simulink model "cv_model_50M"  (R2023a)
settings: Solver=ode23t  StartTime=0  StopTime=5040  FixedStep=0.0005  MaxStep=.01  RelTol=1e-4
model workspace (MAT data in the model file):
  test = 0
values from neighbouring files (symbols this model uses):
  A_cheb_09_1 = [-9.45889157397 1 0 0 0 0 0 0 0 -116.684730988 0 1 ... (81 elements, 9x9)]    [input_reflex_filters.mat]
  B_cheb_09_1 = [1 0 0 0 0 0 0 0 0]    [input_reflex_filters.mat]
  C_cheb_09_1 = [0 0 0 0 0 0 0 0 151338.279895]    [input_reflex_filters.mat]
libraries: SignalEditorBlockLib x4, simulink_extras x2
(part 3 of 3)

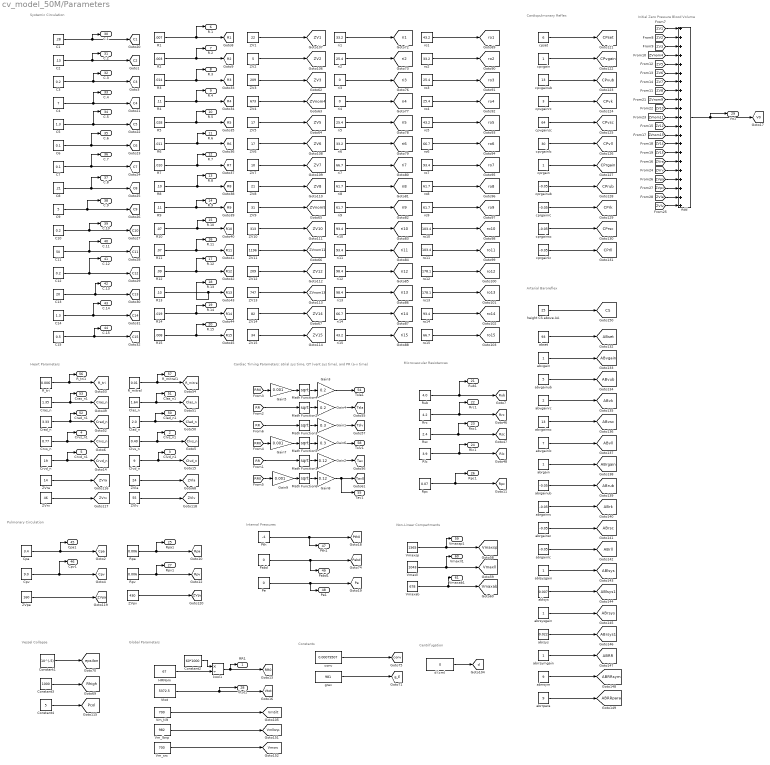
== system cv_model_50M/Parameters ==
  note: Initial Zero Pressure Blood Volume
  note: Cardiopulmonary Reflex
  note: Centrifugation
  note: Constants
  note: Vessel Collapse
  note: Non-Linear Compartments
  note: Heart Parameters
  note: Cardiac Timing Parameters: atrial sys time, QT (vent sys time), and PR (a-v time)
  note: Internal Pressures
  note: Pulmonary Circulation
  note: Microvascular Resistances
  note: Global Parameters
  note: Systemic Circulation
  note: Arterial Baroreflex
  Add : Sum  Inputs=+++++++++++++++++++++
  C1 : Constant  Value=.28
  C10 : Constant  Value=0.2
  C11 : Constant  Value=50
  C12 : Constant  Value=0.2
  C13 : Constant  Value=20
  C14 : Constant  Value=1.3
  C15 : Constant  Value=0.5
  C2 : Constant  Value=.13
  C3 : Constant  Value=0.2
  C4 : Constant  Value=7
  C5 : Constant  Value=1.3
  C6 : Constant  Value=0.1
  C7 : Constant  Value=0.1
  C8 : Constant  Value=.21
  C9 : Constant  Value=5
  Clad_n : Constant  Value=2.0
  Clas_n : Constant  Value=1.64
  Clvd_n : Constant  Value=9
  Clvs_n : Constant  Value=0.40
  Constant1 : Constant  Value=10^(-5)
  Constant2 : Constant  Value=60*1000
  Constant3 : Constant  Value=1000
  Constant4 : Constant  Value=5
  Cpa : Constant  Value=3.4
  Cpv : Constant  Value=9.0
  Crad_n : Constant  Value=3.33
  Cras_n : Constant  Value=1.35
  Crvd_n : Constant  Value=19
  Crvs_n : Constant  Value=0.77
  Gain1 : Gain  Gain=0.3
  Gain2 : Gain  Gain=0.12
  Gain3 : Gain  Gain=0.2
  Gain4 : Gain  Gain=0.2
  Gain5 : Gain  Gain=0.001
  Gain6 : Gain  Gain=0.3
  Gain7 : Gain  Gain=0.001
  Gain8 : Gain  Gain=0.12
  Gain9 : Gain  Gain=0.001
  HRNom : Constant  Value=67
  Math Function{1..6} (6 alike) : Math  Operator=sqrt  SignedPower=on
  Pabd : Constant  Value=0
  Pe : Constant  Value=0
  Pth : Constant  Value=-4
  R1 : Constant  Value=.007
  R10 : Constant  Value=.07
  R11 : Constant  Value=.07
  R12 : Constant  Value=.09
  R13 : Constant  Value=.10
  R14 : Constant  Value=.019
  R15 : Constant  Value=.008
  R2 : Constant  Value=.003
  R3 : Constant  Value=.014
  R4 : Constant  Value=.11
  R5 : Constant  Value=.028
  R6 : Constant  Value=.011
  R7 : Constant  Value=.010
  R8 : Constant  Value=.10
  R9 : Constant  Value=.11
  R_mitral : Constant  Value=0.01
  R_tri : Constant  Value=0.006
  Rlc : Constant  Value=3.9
  Rpa : Constant  Value=0.006
  Rpc : Constant  Value=0.07
  Rpv : Constant  Value=0.006
  Rrc : Constant  Value=4.2
  Rsc : Constant  Value=2.4
  Rub : Constant  Value=4.0
  Vm_lbnp : Constant  Value=982
  Vm_src : Constant  Value=700
  Vm_tilt : Constant  Value=700
  Vmaxab : Constant  Value=678
  Vmaxll : Constant  Value=1043
  Vmaxsp : Constant  Value=1565
  Vtot : Constant  Value=5372.5
  ZV1 : Constant  Value=22
  ZV10 : Constant  Value=313
  ZV11 : Constant  Value=1196
  ZV12 : Constant  Value=209
  ZV13 : Constant  Value=747
  ZV14 : Constant  Value=82
  ZV15 : Constant  Value=34
  ZV2 : Constant  Value=5
  ZV3 : Constant  Value=209
  ZV4 : Constant  Value=673
  ZV5 : Constant  Value=17
  ZV6 : Constant  Value=17
  ZV7 : Constant  Value=10
  ZV8 : Constant  Value=21
  ZV9 : Constant  Value=31
  ZVla : Constant  Value=24
  ZVlv : Constant  Value=55
  ZVpa : Constant  Value=160
  ZVpv : Constant  Value=430
  ZVra : Constant  Value=14
  ZVrv : Constant  Value=46
  ablsys : Constant  Value=0.007
  ablsysgain : Constant
  abrgain : Constant
  abrgainlc : Constant  Value=-0.05
  abrgainrc : Constant  Value=-0.05
  abrgainsc : Constant  Value=-0.05
  abrgainub : Constant  Value=-0.05
  abrrpara : Constant  Value=9
  abrrsym : Constant  Value=9
  abrrsymgain : Constant
  abrsys : Constant  Value=0.022
  abrsysgain : Constant
  abset : Constant  Value=93
  abvgain : Constant
  abvgainlc : Constant  Value=7
  abvgainrc : Constant  Value=2
  abvgainsc : Constant  Value=13
  abvgainub : Constant  Value=5
  conv : Constant  Value=0.00079507
  cprgain : Constant
  cprgainlc : Constant  Value=-0.05
  cprgainrc : Constant  Value=-0.05
  cprgainsc : Constant  Value=-0.05
  cprgainub : Constant  Value=-0.05
  cpset : Constant  Value=6
  cpvgain : Constant
  cpvgainlc : Constant  Value=30
  cpvgainrc : Constant  Value=3
  cpvgainsc : Constant  Value=64
  cpvgainub : Constant  Value=13
  d (cm) : Constant  Value=0
  grav : Constant  Value=981
  height CS above AA : Constant  Value=25
  kool1 : Product  Inputs=*/  InputSameDT=on  SaturateOnIntegerOverflow=on  OutDataTypeStr=Inherit: Same as first input
  ri1 : Constant  Value=33.2
  ri10 : Constant  Value=93.4
  ri11 : Constant  Value=93.4
  ri12 : Constant  Value=98.4
  ri13 : Constant  Value=98.4
  ri14 : Constant  Value=66.7
  ri15 : Constant  Value=43.2
  ri2 : Constant  Value=25.4
  ri3 : Constant  Value=0
  ri4 : Constant  Value=0
  ri5 : Constant  Value=25.4
  ri6 : Constant  Value=33.2
  ri7 : Constant  Value=66.7
  ri8 : Constant  Value=61.7
  ri9 : Constant  Value=61.7
  ro1 : Constant  Value=43.2
  ro10 : Constant  Value=103.4
  ro11 : Constant  Value=103.4
  ro12 : Constant  Value=178.1
  ro13 : Constant  Value=178.1
  ro14 : Constant  Value=93.4
  ro15 : Constant  Value=66.7
  ro2 : Constant  Value=33.2
  ro3 : Constant  Value=25.4
  ro4 : Constant  Value=25.4
  ro5 : Constant  Value=43.2
  ro6 : Constant  Value=66.7
  ro7 : Constant  Value=93.4
  ro8 : Constant  Value=61.7
  ro9 : Constant  Value=61.7
  RR1 : Outport
  Clvs_n1 : Outport  Port=2
  Clvd_n1 : Outport  Port=3
  Crvs_n1 : Outport  Port=4
  Crvd_n1 : Outport  Port=5
  R.1 : Outport  Port=6
  R.2 : Outport  Port=7
  R.3 : Outport  Port=8
  R.4 : Outport  Port=9
  R.5 : Outport  Port=10
  R.6 : Outport  Port=11
  R.7 : Outport  Port=12
  R.8 : Outport  Port=13
  R.9 : Outport  Port=14
  R.10 : Outport  Port=15
  R.11 : Outport  Port=16
  R.12 : Outport  Port=17
  R.13 : Outport  Port=18
  R.14 : Outport  Port=19
  R.15 : Outport  Port=20
  Rub1 : Outport  Port=21
  Rrc1 : Outport  Port=22
  Rsc1 : Outport  Port=23
  Rlc1 : Outport  Port=24
  Rpa1 : Outport  Port=25
  Rpc1 : Outport  Port=26
  Rpv1 : Outport  Port=27
  Vtot1 : Outport  Port=28
  Vo1 : Outport  Port=29
  C.1 : Outport  Port=30
  C.2 : Outport  Port=31
  C.3 : Outport  Port=32
  C.4 : Outport  Port=33
  C.5 : Outport  Port=34
  C.6 : Outport  Port=35
  C.7 : Outport  Port=36
  C.8 : Outport  Port=37
  C.9 : Outport  Port=38
  C.10 : Outport  Port=39
  C.11 : Outport  Port=40
  C.12 : Outport  Port=41
  C.13 : Outport  Port=42
  C.14 : Outport  Port=43
  C.15 : Outport  Port=44
  Cpa1 : Outport  Port=45
  Cpv1 : Outport  Port=46
  Pth1 : Outport  Port=47
  Pe1 : Outport  Port=48
  Pabd1 : Outport  Port=49
  Clad_n1 : Outport  Port=50
  Clas_n1 : Outport  Port=51
  Crad_n1 : Outport  Port=52
  Cras_n1 : Outport  Port=53
  Tsla1 : Outport  Port=54
  Tav1 : Outport  Port=55
  R_tri1 : Outport  Port=56
  R_mitral1 : Outport  Port=57
  Tslv1 : Outport  Port=58
  Vmaxsp1 : Outport  Port=59
  Vmaxll1 : Outport  Port=60
  Vmaxab1 : Outport  Port=61
  tag scope: ABRR=global, ABRRpara=global, ABRRsym=global, ABlsys1=global, ABlsys=global, ABrgain=global, ABrk=global, ABrll=global, ABrsc=global, ABrsys1=global, ABrsys=global, ABrub=global, ABset=global, ABvgain=global, ABvk=global, ABvll=global, ABvsc=global, ABvub=global, C10=global, C11=global, C12=global, C13=global, C14=global, C15=global, C1=global, C2=global, C3=global, C4=global, C5=global, C6=global, C7=global, C8=global, C9=global, CPrgain=global, CPrk=global, CPrll=global, CPrsc=global, CPrub=global, CPset=global, CPvgain=global, CPvk=global, CPvll=global, CPvsc=global, CPvub=global, CS=global, Clad_n=global, Clas_n=global, Clvd_n=global, Clvs_n=global, Cpa=global, Cpv=global, Crad_n=global, Cras_n=global, Crvd_n=global, Crvs_n=global, Pabd=global, Pcol=global, Pe=global, Pth0=global, R10=global, R11=global, R12=global, R13=global, R14=global, R15=global, R1=global, R2=global, R3=global, R4=global, R5=global, R6=global, R7=global, R8=global, R9=global, RR0=global, R_mitral=global, R_tri=global, Rhigh=global, Rlc=global, Rpa=global, Rpc=global, Rpv=global, Rrc=global, Rsc=global, Rub=global, Tav0=global, Tav=global, Tsla=global, Tslv=global, V0=global, Vmaxab=global, Vmaxll=global, Vmaxsp=global, Vmlbnp=global, Vmsrc=global, Vmtilt=global, Vtot=global, ZV10=global, ZV12=global, ZV14=global, ZV15=global, ZV1=global, ZV2=global, ZV3=global, ZV5=global, ZV6=global, ZV7=global, ZV8=global, ZVla=global, ZVlv=global, ZVnom11=global, ZVnom13=global, ZVnom4=global, ZVnom9=global, ZVpa=global, ZVpv=global, ZVra=global, ZVrv=global, conv=global, d=global, epsilon=global, g_E=global, ri10=global, ri11=global, ri12=global, ri13=global, ri14=global, ri15=global, ri1=global, ri2=global, ri3=global, ri4=global, ri5=global, ri6=global, ri7=global, ri8=global, ri9=global, ro10=global, ro11=global, ro12=global, ro13=global, ro14=global, ro15=global, ro1=global, ro2=global, ro3=global, ro4=global, ro5=global, ro6=global, ro7=global, ro8=global, ro9=global
  wires:
  Cpa/1 -> [Cpa], Cpa1/1
  Cpv/1 -> [Cpv], Cpv1/1
  Clvs_n/1 -> Clvs_n1/1, [Clvs_n]
  Crvs_n/1 -> [Crvs_n], Crvs_n1/1
  Rpa/1 -> Rpa1/1, [Rpa]
  Rpc/1 -> [Rpc], Rpc1/1
  Rpv/1 -> Rpv1/1, [Rpv]
  Crvd_n/1 -> [Crvd_n], Crvd_n1/1
  Clvd_n/1 -> Clvd_n1/1, [Clvd_n]
  Add/1 -> Vo1/1, [V0]
  Pth/1 -> Pth1/1, [Pth0]
  C1/1 -> [C1], C.1/1
  C2/1 -> [C2], C.2/1
  C3/1 -> [C3], C.3/1
  C4/1 -> [C4], C.4/1
  C5/1 -> C.5/1, [C5]
  C6/1 -> C.6/1, [C6]
  C7/1 -> C.7/1, [C7]
  C8/1 -> [C8], C.8/1
  C9/1 -> C.9/1, [C9]
  C10/1 -> C.10/1, [C10]
  C11/1 -> C.11/1, [C11]
  C12/1 -> C.12/1, [C12]
  C13/1 -> [C13], C.13/1
  C14/1 -> [C14], C.14/1
  R1/1 -> [R1], R.1/1
  R2/1 -> [R2], R.2/1
  R3/1 -> [R3], R.3/1
  R4/1 -> [R4], R.4/1
  R5/1 -> [R5], R.5/1
  R6/1 -> [R6], R.6/1
  R7/1 -> [R7], R.7/1
  R8/1 -> [R8], R.8/1
  R9/1 -> [R9], R.9/1
  R10/1 -> [R10], R.10/1
  R11/1 -> [R11], R.11/1
  R12/1 -> [R12], R.12/1
  R13/1 -> R.13/1, [R13]
  R14/1 -> [R14], R.14/1
  R15/1 -> [R15], R.15/1
  Rub/1 -> Rub1/1, [Rub]
  Rrc/1 -> [Rrc], Rrc1/1
  Rsc/1 -> [Rsc], Rsc1/1
  Rlc/1 -> [Rlc], Rlc1/1
  C15/1 -> C.15/1, [C15]
  Pe/1 -> Pe1/1, [Pe]
  Cras_n/1 -> [Cras_n], Cras_n1/1
  Clad_n/1 -> [Clad_n], Clad_n1/1
  Crad_n/1 -> Crad_n1/1, [Crad_n]
  R_tri/1 -> [R_tri], R_tri1/1
  R_mitral/1 -> [R_mitral], R_mitral1/1
  Math Function3/1 -> Gain1/1
  [RR] -> Math Function3/1
  Gain1/1 -> [Tslv]
  Gain2/1 -> [Tav]
  Math Function2/1 -> Gain4/1
  [RR] -> Math Function2/1
  Gain4/1 -> [Tsla]
  Math Function1/1 -> Gain2/1
  [RR] -> Math Function1/1
  Clas_n/1 -> [Clas_n], Clas_n1/1
  Vmaxsp/1 -> [Vmaxsp], Vmaxsp1/1
  Vmaxll/1 -> Vmaxll1/1, [Vmaxll]
  Vmaxab/1 -> Vmaxab1/1, [Vmaxab]
  Math Function4/1 -> Gain3/1
  [RR0] -> Gain5/1
  Gain5/1 -> Math Function4/1
  Gain3/1 -> Tsla1/1
  Math Function5/1 -> Gain6/1
  [RR0] -> Gain7/1
  Gain7/1 -> Math Function5/1
  Gain6/1 -> Tslv1/1
  Math Function6/1 -> Gain8/1
  [RR0] -> Gain9/1
  Gain9/1 -> Math Function6/1
  Gain8/1 -> Tav1/1, [Tav0]
  ZV3/1 -> [ZV3]
  ZV4/1 -> [ZVnom4]
  ZV5/1 -> [ZV5]
  ZV9/1 -> [ZVnom9]
  ZV11/1 -> [ZVnom11]
  ZV14/1 -> [ZV14]
  ZVla/1 -> [ZVla]
  Constant3/1 -> [Rhigh]
  Constant1/1 -> [epsilon]
  Vtot/1 -> [Vtot], Vtot1/1
  Pabd/1 -> [Pabd], Pabd1/1
  conv/1 -> [conv]
  Constant2/1 -> kool1/1
  HRNom/1 -> kool1/2
  kool1/1 -> [RR0], RR1/1
  ri1/1 -> [ri1]
  ri2/1 -> [ri2]
  ri3/1 -> [ri3]
  ri4/1 -> [ri4]
  ri5/1 -> [ri5]
  ri6/1 -> [ri6]
  ri7/1 -> [ri7]
  ri8/1 -> [ri8]
  ri9/1 -> [ri9]
  ri10/1 -> [ri10]
  ri11/1 -> [ri11]
  ri12/1 -> [ri12]
  ri13/1 -> [ri13]
  ri14/1 -> [ri14]
  ri15/1 -> [ri15]
  ro1/1 -> [ro1]
  ro2/1 -> [ro2]
  ro3/1 -> [ro3]
  ro4/1 -> [ro4]
  ro5/1 -> [ro5]
  ro6/1 -> [ro6]
  ro7/1 -> [ro7]
  ro8/1 -> [ro8]
  ro9/1 -> [ro9]
  ro10/1 -> [ro10]
  ro11/1 -> [ro11]
  ro12/1 -> [ro12]
  ro13/1 -> [ro13]
  ro14/1 -> [ro14]
  ro15/1 -> [ro15]
  d (cm)/1 -> [d]
  Vm_tilt/1 -> [Vmtilt]
  grav/1 -> [g_E]
  ZV2/1 -> [ZV2]
  ZV1/1 -> [ZV1]
  ZV6/1 -> [ZV6]
  ZV7/1 -> [ZV7]
  ZV8/1 -> [ZV8]
  ZV10/1 -> [ZV10]
  ZV12/1 -> [ZV12]
  ZV13/1 -> [ZVnom13]
  ZV15/1 -> [ZV15]
  Constant4/1 -> [Pcol]
  ZVra/1 -> [ZVra]
  ZVrv/1 -> [ZVrv]
  ZVlv/1 -> [ZVlv]
  ZVpa/1 -> [ZVpa]
  ZVpv/1 -> [ZVpv]
  cpset/1 -> [CPset]
  cpvgain/1 -> [CPvgain]
  cpvgainub/1 -> [CPvub]
  cpvgainrc/1 -> [CPvk]
  cpvgainsc/1 -> [CPvsc]
  cpvgainlc/1 -> [CPvll]
  cprgain/1 -> [CPrgain]
  cprgainub/1 -> [CPrub]
  cprgainrc/1 -> [CPrk]
  cprgainsc/1 -> [CPrsc]
  cprgainlc/1 -> [CPrll]
  abrgainub/1 -> [ABrub]
  abrgainrc/1 -> [ABrk]
  abvgainlc/1 -> [ABvll]
  abset/1 -> [ABset]
  abvgainrc/1 -> [ABvk]
  abvgainub/1 -> [ABvub]
  abvgainsc/1 -> [ABvsc]
  abvgain/1 -> [ABvgain]
  abrgain/1 -> [ABrgain]
  abrgainlc/1 -> [ABrll]
  abrgainsc/1 -> [ABrsc]
  ablsysgain/1 -> [ABlsys]
  ablsys/1 -> [ABlsys1]
  abrsysgain/1 -> [ABrsys]
  abrsys/1 -> [ABrsys1]
  abrrpara/1 -> [ABRRpara]
  abrrsym/1 -> [ABRRsym]
  abrrsymgain/1 -> [ABRR]
  height CS above AA/1 -> [CS]
  [ZV1] -> Add/1
  [ZV2] -> Add/2
  [ZV3] -> Add/3
  [ZVnom4] -> Add/4
  [ZV5] -> Add/5
  [ZV6] -> Add/6
  [ZV7] -> Add/7
  [ZV8] -> Add/8
  [ZVnom9] -> Add/9
  [ZV10] -> Add/10
  [ZVnom11] -> Add/11
  [ZV12] -> Add/12
  [ZVnom13] -> Add/13
  [ZV14] -> Add/14
  [ZV15] -> Add/15
  [ZVra] -> Add/16
  [ZVrv] -> Add/17
  [ZVpa] -> Add/18
  [ZVpv] -> Add/19
  [ZVla] -> Add/20
  [ZVlv] -> Add/21
  Vm_lbnp/1 -> [Vmlbnp]
  Vm_src/1 -> [Vmsrc]

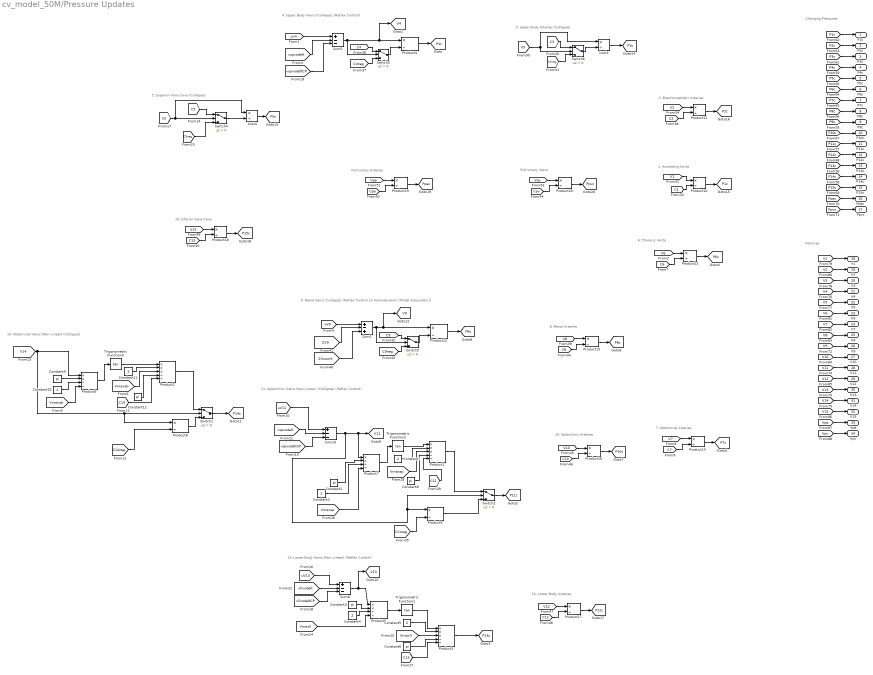
== system cv_model_50M/Pressure Updates ==
  note: 11: Splanchnic Veins (Non-Linear) (Collapse) (Reflex Control)
  note: 14: Abdominal Veins (Non-Linear) (Collapse)
  note: 13: Lower Body Veins (Non-Linear) (Reflex Control)
  note: 10: Splanchnic Arteries
  note: 15: Inferior Vena Cava
  note: 12: Lower Body Arteries
  note: Pulmonary Arteries
  note: Pulmonary Veins
  note: 9: Renal Veins (Collapse) (Reflex Control [in Hemodynamic Model Subsystem])
  note: 8: Renal Arteries
  note: 7: Abdominal Arteries
  note: 6: Thoracic Aorta
  note: 5: Superior Vena Cava (Collapse)
  note: 4: Upper Body Veins (Collapse) (Reflex Control)
  note: 3: Upper Body Arteries (Collapse)
  note: 2: Brachiocephalic Arteries
  note: 1: Ascending Aorta
  note: Volumes
  note: Changing Pressures
  Constant{1,3,6,8..9,12} (6 alike) : Constant  Value=pi
  Constant{2,4..5,7,10..11} (6 alike) : Constant  Value=2
  Product1 : Product  Inputs=***//  SaturateOnIntegerOverflow=on  OutDataTypeStr=Inherit: Same as first input
  Product{4,8..20} (14 alike) : Product  Inputs=*/  SaturateOnIntegerOverflow=on  OutDataTypeStr=Inherit: Same as first input
  Product2 : Product  Inputs=***//  SaturateOnIntegerOverflow=on  OutDataTypeStr=Inherit: Same as first input
  Product3 : Product  Inputs=***//  SaturateOnIntegerOverflow=on  OutDataTypeStr=Inherit: Same as first input
  Product5 : Product  Inputs=**//  SaturateOnIntegerOverflow=on  OutDataTypeStr=Inherit: Same as first input
  Product6 : Product  Inputs=**//  SaturateOnIntegerOverflow=on  OutDataTypeStr=Inherit: Same as first input
  Product7 : Product  Inputs=**//  SaturateOnIntegerOverflow=on  OutDataTypeStr=Inherit: Same as first input
  Sum1 : Sum  Inputs=+-+  InputSameDT=on  SaturateOnIntegerOverflow=on  OutDataTypeStr=Inherit: Same as first input
  Sum10 : Sum  Inputs=+--  InputSameDT=on  SaturateOnIntegerOverflow=on  OutDataTypeStr=Inherit: Same as first input
  Sum5 : Sum  Inputs=+--  InputSameDT=on  SaturateOnIntegerOverflow=on  OutDataTypeStr=Inherit: Same as first input
  Sum8 : Sum  Inputs=+--  InputSameDT=on  SaturateOnIntegerOverflow=on  OutDataTypeStr=Inherit: Same as first input
  Switch{1..6} (6 alike) : Switch  Criteria=u2 > Threshold
  Trigonometric Function1 : Trigonometry  Operator=tan
  Trigonometric Function2 : Trigonometry  Operator=tan
  Trigonometric Function3 : Trigonometry  Operator=tan
  kool3 : Product  Inputs=*/  InputSameDT=on  SaturateOnIntegerOverflow=on  OutDataTypeStr=Inherit: Same as first input
  kool4 : Product  Inputs=*/  InputSameDT=on  SaturateOnIntegerOverflow=on  OutDataTypeStr=Inherit: Same as first input
  P1c : Outport
  P2c : Outport  Port=2
  P3c : Outport  Port=3
  P4c : Outport  Port=4
  P5c : Outport  Port=5
  P6c : Outport  Port=6
  P7c : Outport  Port=7
  P8c : Outport  Port=8
  P9c : Outport  Port=9
  P10c : Outport  Port=10
  P11c : Outport  Port=11
  P12c : Outport  Port=12
  P13c : Outport  Port=13
  P14c : Outport  Port=14
  P15c : Outport  Port=15
  Ppac : Outport  Port=16
  Ppvc : Outport  Port=17
  V1 : Outport  Port=18
  V2 : Outport  Port=19
  V3 : Outport  Port=20
  V4 : Outport  Port=21
  V5 : Outport  Port=22
  V6 : Outport  Port=23
  V7 : Outport  Port=24
  V8 : Outport  Port=25
  V9 : Outport  Port=26
  V10 : Outport  Port=27
  V11 : Outport  Port=28
  V12 : Outport  Port=29
  V13 : Outport  Port=30
  V14 : Outport  Port=31
  V15 : Outport  Port=32
  Vpa : Outport  Port=33
  Vpv : Outport  Port=34
  tag scope: P10c=global, P11c=global, P12c=global, P13c=global, P14c=global, P15c=global, P1c=global, P2c=global, P3c=global, P4c=global, P5c=global, P6c=global, P7c=global, P8c=global, P9c=global, Ppac=global, Ppvc=global, V11=global, V13=global, V4=global, V9=global
  wires:
  Product3/1 -> [P13c]
  [vllvodelt] -> Sum8/2
  [vllvodeltCP] -> Sum8/3
  Sum8/1 -> [V13], Product6/1
  [uV13] -> Sum8/1
  Constant3/1 -> Product6/2
  Constant4/1 -> Product6/3
  [Vmaxll] -> Product6/4
  Product6/1 -> Trigonometric Function1/1
  Trigonometric Function1/1 -> Product3/1
  Constant5/1 -> Product3/2
  [Vmaxll] -> Product3/3
  Constant6/1 -> Product3/4
  [C13] -> Product3/5
  [vspvodelt] -> Sum10/2
  [vspvodeltCP] -> Sum10/3
  Sum10/1 -> Product9/1, Switch2/2, Product7/1, [V11]
  [uV11] -> Sum10/1
  [vupvodeltCP] -> Sum5/3
  [uV4] -> Sum5/1
  Sum5/1 -> Switch3/2, Product4/1, [V4]
  Product4/1 -> [P4c]
  [ZV9] -> Sum1/2
  [ZVnom9] -> Sum1/3
  [uV9] -> Sum1/1
  Sum1/1 -> Switch5/2, Product12/1, [V9]
  Product12/1 -> [P9c]
  [C9] -> Switch5/1
  [C9neg] -> Switch5/3
  Switch5/1 -> Product12/2
  [C4] -> Switch3/1
  [C4neg] -> Switch3/3
  Switch3/1 -> Product4/2
  Product1/1 -> Switch2/1
  Constant1/1 -> Product7/2
  Constant2/1 -> Product7/3
  [Vmaxsp] -> Product7/4
  Product7/1 -> Trigonometric Function2/1
  Trigonometric Function2/1 -> Product1/1
  Constant7/1 -> Product1/2
  [Vmaxsp] -> Product1/3
  Constant8/1 -> Product1/4
  [C11] -> Product1/5
  Switch2/1 -> [P11c]
  [C11neg] -> Product9/2
  Product9/1 -> Switch2/3
  [V14] -> Product8/1, Switch1/2, Product5/1
  Product2/1 -> Switch1/1
  Constant9/1 -> Product5/2
  Constant10/1 -> Product5/3
  [Vmaxab] -> Product5/4
  Product5/1 -> Trigonometric Function3/1
  Trigonometric Function3/1 -> Product2/1
  Constant11/1 -> Product2/2
  [Vmaxab] -> Product2/3
  Constant12/1 -> Product2/4
  [C14] -> Product2/5
  Switch1/1 -> [P14c]
  [C14neg] -> Product8/2
  Product8/1 -> Switch1/3
  [V5] -> Switch4/2, kool4/1
  [C5] -> Switch4/1
  [C5neg] -> Switch4/3
  Switch4/1 -> kool4/2
  kool4/1 -> [P5c]
  [V3] -> Switch6/2, kool3/1
  [C3] -> Switch6/1
  [C3neg] -> Switch6/3
  Switch6/1 -> kool3/2
  kool3/1 -> [P3c]
  [V1] -> Product10/1
  [C1] -> Product10/2
  Product10/1 -> [P1c]
  [V2] -> Product11/1
  [C2] -> Product11/2
  Product11/1 -> [P2c]
  [V6] -> Product13/1
  [C6] -> Product13/2
  Product13/1 -> [P6c]
  [V7] -> Product14/1
  [C7] -> Product14/2
  Product14/1 -> [P7c]
  [V8] -> Product15/1
  [C8] -> Product15/2
  Product15/1 -> [P8c]
  [V10] -> Product16/1
  [C10] -> Product16/2
  Product16/1 -> [P10c]
  [V12] -> Product17/1
  [C12] -> Product17/2
  Product17/1 -> [P12c]
  [V15] -> Product18/1
  [C15] -> Product18/2
  Product18/1 -> [P15c]
  [Vpa] -> Product19/1
  [Cpa] -> Product19/2
  Product19/1 -> [Ppac]
  [Vpv] -> Product20/1
  [Cpv] -> Product20/2
  Product20/1 -> [Ppvc]
  [P1c] -> P1c/1
  [P2c] -> P2c/1
  [P3c] -> P3c/1
  [P4c] -> P4c/1
  [P5c] -> P5c/1
  [P6c] -> P6c/1
  [P7c] -> P7c/1
  [P8c] -> P8c/1
  [P9c] -> P9c/1
  [P10c] -> P10c/1
  [P11c] -> P11c/1
  [P12c] -> P12c/1
  [P13c] -> P13c/1
  [P14c] -> P14c/1
  [P15c] -> P15c/1
  [Ppac] -> Ppac/1
  [Ppvc] -> Ppvc/1
  [Vpv] -> Vpv/1
  [Vpa] -> Vpa/1
  [V4] -> V4/1
  [V15] -> V15/1
  [V12] -> V12/1
  [V13] -> V13/1
  [V14] -> V14/1
  [V2] -> V2/1
  [V1] -> V1/1
  [V10] -> V10/1
  [V11] -> V11/1
  [V9] -> V9/1
  [V7] -> V7/1
  [V6] -> V6/1
  [V5] -> V5/1
  [V8] -> V8/1
  [V3] -> V3/1
  [vupvodelt] -> Sum5/2

== system cv_model_50M/RA Cap. ==
  note: 3/2*Tsla > t
  note: Tsla < t < 3/2*Tsla
  note: 0 < t < Tsla
  Constant : Constant
  Constant1 : Constant  Value=pi
  Constant2 : Constant
  Constant3 : Constant  Value=2*pi
  Gain : Gain  Gain=0.5
  Gain1 : Gain  Gain=1.5
  Gain2 : Gain  Gain=0.5
  Math Function{,1..7} (8 alike) : Math  Operator=reciprocal  SignedPower=on
  Sum{1..3,5..6,9} (6 alike) : Sum  Inputs=+-  InputSameDT=on  SaturateOnIntegerOverflow=on  OutDataTypeStr=Inherit: Same as first input
  Sum4 : Sum  InputSameDT=on  SaturateOnIntegerOverflow=on  OutDataTypeStr=Inherit: Same as first input
  Sum7 : Sum  InputSameDT=on  SaturateOnIntegerOverflow=on  OutDataTypeStr=Inherit: Same as first input
  Sum8 : Sum  InputSameDT=on  SaturateOnIntegerOverflow=on  OutDataTypeStr=Inherit: Same as first input
  Switch1 : Switch
  Switch2 : Switch
  Trigonometric Function : Trigonometry  Operator=cos
  Trigonometric Function1 : Trigonometry  Operator=cos
  mult : Product  Inputs=**
  mult1 : Product  Inputs=**/
  mult3 : Product  Inputs=**
  mult4 : Product  Inputs=**/
  Cra : Outport
  tag scope: Cra=global
  wires:
  [Tsla] -> Sum9/2
  Sum9/1 -> Switch1/2
  [Cras_n] -> Math Function/1
  Sum3/1 -> Gain/1
  Gain/1 -> mult/1
  Constant/1 -> Sum1/1
  Trigonometric Function/1 -> Sum1/2
  Constant1/1 -> mult1/1
  mult1/1 -> Trigonometric Function/1
  [Tsla] -> mult1/3
  Sum1/1 -> mult/2
  [t] -> mult1/2
  mult/1 -> Sum7/1
  Math Function/1 -> Sum3/1
  [Crad_n] -> Math Function1/1
  Math Function1/1 -> Sum3/2
  [Crad_n] -> Math Function2/1
  Math Function2/1 -> Sum7/2
  Sum7/1 -> Switch1/3
  [t] -> Sum2/1
  [Tsla] -> Gain1/1
  Gain1/1 -> Sum2/2
  Switch2/1 -> Switch1/1
  Sum2/1 -> Switch2/2
  Sum6/1 -> Gain2/1
  Gain2/1 -> mult3/1
  Constant2/1 -> Sum4/1
  Trigonometric Function1/1 -> Sum4/2
  Constant3/1 -> mult4/1
  mult4/1 -> Trigonometric Function1/1
  [Tsla] -> mult4/3
  Sum4/1 -> mult3/2
  Sum5/1 -> mult4/2
  mult3/1 -> Sum8/1
  [Tsla] -> Sum5/2
  [Cras_n] -> Math Function3/1
  Math Function3/1 -> Sum6/1
  [Crad_n] -> Math Function4/1
  Math Function4/1 -> Sum6/2
  [Crad_n] -> Math Function5/1
  Math Function5/1 -> Sum8/2
  [t] -> Sum5/1
  [t] -> Sum9/1
  Sum8/1 -> Switch2/3
  [Crad_n] -> Math Function6/1
  Math Function6/1 -> Switch2/1
  Switch1/1 -> Math Function7/1
  Math Function7/1 -> [Cra], Cra/1

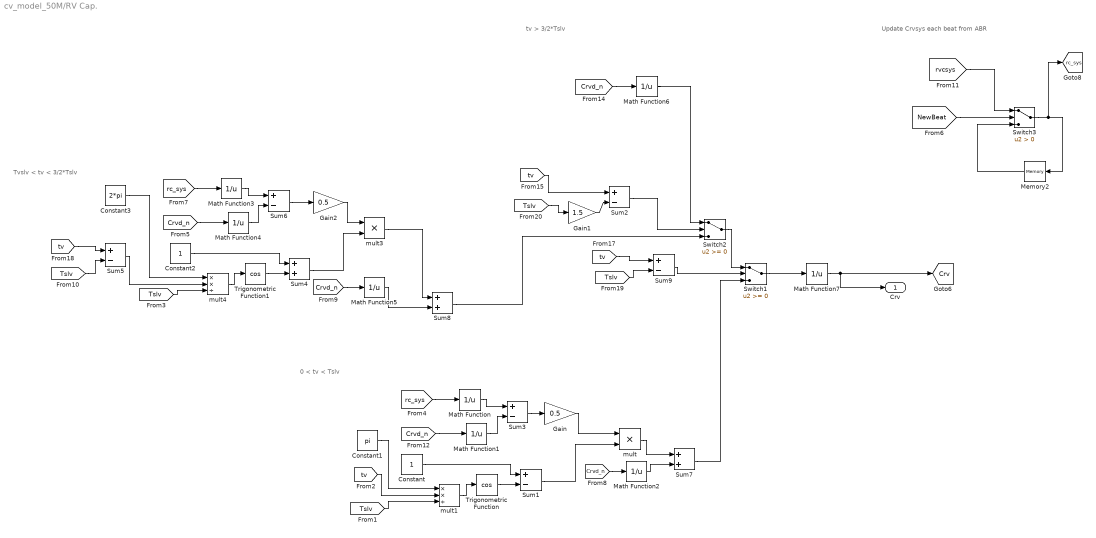
== system cv_model_50M/RV Cap. ==
  note: Update Crvsys each beat from ABR
  note: tv > 3/2*Tslv
  note: Tvslv < tv < 3/2*Tslv
  note: 0 < tv < Tslv
  Constant : Constant
  Constant1 : Constant  Value=pi
  Constant2 : Constant
  Constant3 : Constant  Value=2*pi
  Gain : Gain  Gain=0.5
  Gain1 : Gain  Gain=1.5
  Gain2 : Gain  Gain=0.5
  Math Function{,1..7} (8 alike) : Math  Operator=reciprocal  SignedPower=on
  Memory2 : Memory  InitialCondition=1.2  InheritSampleTime=on
  Sum{1..3,5..6,9} (6 alike) : Sum  Inputs=+-  InputSameDT=on  SaturateOnIntegerOverflow=on  OutDataTypeStr=Inherit: Same as first input
  Sum4 : Sum  InputSameDT=on  SaturateOnIntegerOverflow=on  OutDataTypeStr=Inherit: Same as first input
  Sum7 : Sum  InputSameDT=on  SaturateOnIntegerOverflow=on  OutDataTypeStr=Inherit: Same as first input
  Sum8 : Sum  InputSameDT=on  SaturateOnIntegerOverflow=on  OutDataTypeStr=Inherit: Same as first input
  Switch1 : Switch
  Switch2 : Switch
  Switch3 : Switch  Criteria=u2 > Threshold
  Trigonometric Function : Trigonometry  Operator=cos
  Trigonometric Function1 : Trigonometry  Operator=cos
  mult : Product  Inputs=**
  mult1 : Product  Inputs=**/
  mult3 : Product  Inputs=**
  mult4 : Product  Inputs=**/
  Crv : Outport
  tag scope: Crv=global, rc_sys=global
  wires:
  [Tslv] -> Sum9/2
  Sum9/1 -> Switch1/2
  [rc_sys] -> Math Function/1
  Sum3/1 -> Gain/1
  Gain/1 -> mult/1
  Constant/1 -> Sum1/1
  Trigonometric Function/1 -> Sum1/2
  Constant1/1 -> mult1/1
  mult1/1 -> Trigonometric Function/1
  [Tslv] -> mult1/3
  Sum1/1 -> mult/2
  [tv] -> mult1/2
  mult/1 -> Sum7/1
  Math Function/1 -> Sum3/1
  [Crvd_n] -> Math Function1/1
  Math Function1/1 -> Sum3/2
  [Crvd_n] -> Math Function2/1
  Math Function2/1 -> Sum7/2
  Sum7/1 -> Switch1/3
  [tv] -> Sum2/1
  [Tslv] -> Gain1/1
  Gain1/1 -> Sum2/2
  Switch2/1 -> Switch1/1
  Sum2/1 -> Switch2/2
  Sum6/1 -> Gain2/1
  Gain2/1 -> mult3/1
  Constant2/1 -> Sum4/1
  Trigonometric Function1/1 -> Sum4/2
  Constant3/1 -> mult4/1
  mult4/1 -> Trigonometric Function1/1
  [Tslv] -> mult4/3
  Sum4/1 -> mult3/2
  Sum5/1 -> mult4/2
  mult3/1 -> Sum8/1
  [Tslv] -> Sum5/2
  [rc_sys] -> Math Function3/1
  Math Function3/1 -> Sum6/1
  [Crvd_n] -> Math Function4/1
  Math Function4/1 -> Sum6/2
  [Crvd_n] -> Math Function5/1
  Math Function5/1 -> Sum8/2
  [tv] -> Sum5/1
  [tv] -> Sum9/1
  Sum8/1 -> Switch2/3
  [Crvd_n] -> Math Function6/1
  Math Function6/1 -> Switch2/1
  Switch1/1 -> Math Function7/1
  Math Function7/1 -> [Crv], Crv/1
  [NewBeat] -> Switch3/2
  [rvcsys] -> Switch3/1
  Switch3/1 -> Memory2/1, [rc_sys]
  Memory2/1 -> Switch3/3

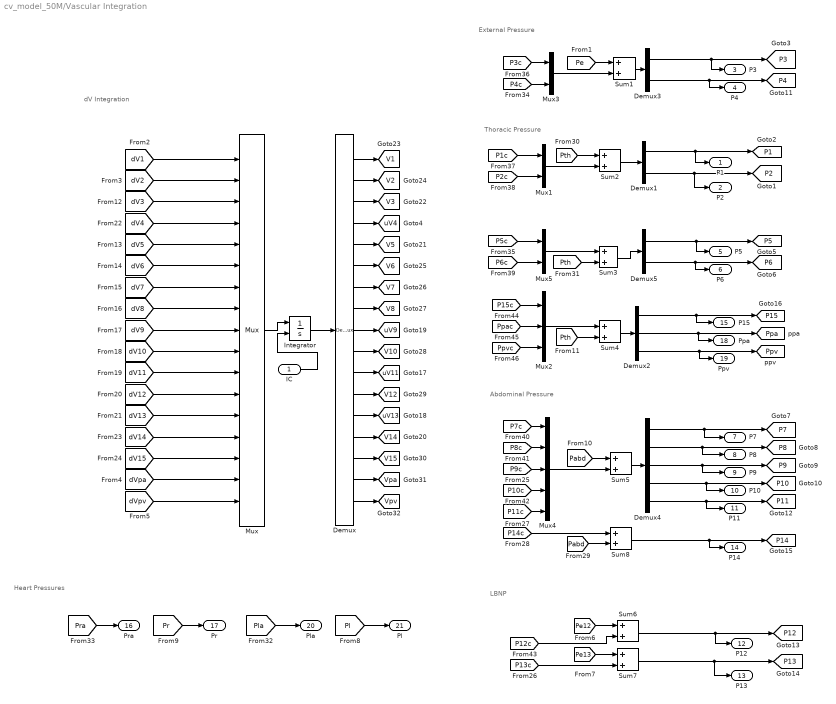
== system cv_model_50M/Vascular Integration ==
  note: Heart Pressures
  note: dV Integration
  note: External Pressure
  note: LBNP
  note: Abdominal Pressure
  note: Thoracic Pressure
  IC : Inport
  Demux : Demux  Outputs=17
      settings: DisplayOption=none
  Demux1 : Demux  Outputs=2
      settings: DisplayOption=none
  Demux2 : Demux  Outputs=3
      settings: DisplayOption=none
  Demux3 : Demux  Outputs=2
      settings: DisplayOption=none
  Demux4 : Demux  Outputs=5
      settings: DisplayOption=none
  Demux5 : Demux  Outputs=2
      settings: DisplayOption=none
  Integrator : Integrator  InitialConditionSource=external  InitialCondition=[113.4187 4.15 24.2091 19.3527]
  Mux : Mux  Inputs=17
  Mux1 : Mux  Inputs=2
  Mux2 : Mux  Inputs=3
  Mux3 : Mux  Inputs=2
  Mux4 : Mux  Inputs=5
  Mux5 : Mux  Inputs=2
  Sum{1..8} (8 alike) : Sum  InputSameDT=on  SaturateOnIntegerOverflow=on  OutDataTypeStr=Inherit: Same as first input
  P1 : Outport
  P2 : Outport  Port=2
  P3 : Outport  Port=3
  P4 : Outport  Port=4
  P5 : Outport  Port=5
  P6 : Outport  Port=6
  P7 : Outport  Port=7
  P8 : Outport  Port=8
  P9 : Outport  Port=9
  P10 : Outport  Port=10
  P11 : Outport  Port=11
  P12 : Outport  Port=12
  P13 : Outport  Port=13
  P14 : Outport  Port=14
  P15 : Outport  Port=15
  Pra : Outport  Port=16
  Pr : Outport  Port=17
  Ppa : Outport  Port=18
  Ppv : Outport  Port=19
  Pla : Outport  Port=20
  Pl : Outport  Port=21
  tag scope: P10=global, P11=global, P12=global, P13=global, P14=global, P15=global, P1=global, P2=global, P3=global, P4=global, P5=global, P6=global, P7=global, P8=global, P9=global, Ppa=global, Ppv=global, V10=global, V12=global, V14=global, V15=global, V1=global, V2=global, V3=global, V5=global, V6=global, V7=global, V8=global, Vpa=global, Vpv=global, uV11=global, uV13=global, uV4=global, uV9=global
  wires:
  [Pl] -> Pl/1
  [Pr] -> Pr/1
  [dV1] -> Mux/1
  [dV2] -> Mux/2
  Demux2/2 -> Ppa/1, [Ppa]
  Demux1/1 -> P1/1, [P1]
  [dVpv] -> Mux/17
  [dVpa] -> Mux/16
  [dV3] -> Mux/3
  [dV4] -> Mux/4
  [dV5] -> Mux/5
  [dV6] -> Mux/6
  [dV7] -> Mux/7
  [dV8] -> Mux/8
  [dV9] -> Mux/9
  [dV10] -> Mux/10
  [dV11] -> Mux/11
  [dV12] -> Mux/12
  [dV13] -> Mux/13
  [dV14] -> Mux/14
  [dV15] -> Mux/15
  Demux1/2 -> [P2], P2/1
  Demux3/1 -> P3/1, [P3]
  Demux3/2 -> [P4], P4/1
  Demux5/1 -> [P5], P5/1
  Demux4/1 -> P7/1, [P7]
  Demux4/2 -> P8/1, [P8]
  Demux4/3 -> [P9], P9/1
  Demux4/4 -> P10/1, [P10]
  Demux4/5 -> P11/1, [P11]
  Demux2/1 -> [P15], P15/1
  Demux2/3 -> Ppv/1, [Ppv]
  Demux5/2 -> P6/1, [P6]
  Integrator/1 -> Demux/1
  Mux/1 -> Integrator/1
  IC/1 -> Integrator/2
  [Pth] -> Sum4/2
  Mux1/1 -> Sum2/2
  Sum2/1 -> Demux1/1
  Sum6/1 -> [P12], P12/1
  Sum7/1 -> [P13], P13/1
  Sum8/1 -> [P14], P14/1
  Mux2/1 -> Sum4/1
  Sum4/1 -> Demux2/1
  [Pth] -> Sum2/1
  Demux/4 -> [uV4]
  Mux3/1 -> Sum1/2
  Sum1/1 -> Demux3/1
  [Pe] -> Sum1/1
  [Pth] -> Sum3/2
  [Pabd] -> Sum5/1
  Mux4/1 -> Sum5/2
  Sum5/1 -> Demux4/1
  Mux5/1 -> Sum3/1
  Sum3/1 -> Demux5/1
  [Pe12] -> Sum6/1
  [Pabd] -> Sum8/2
  [Pla] -> Pla/1
  [Pra] -> Pra/1
  [P4c] -> Mux3/2
  [P11c] -> Mux4/5
  Demux/13 -> [uV13]
  [P13c] -> Sum7/2
  Demux/9 -> [uV9]
  [P9c] -> Mux4/3
  Demux/14 -> [V14]
  [P14c] -> Sum8/1
  [P5c] -> Mux5/1
  Demux/5 -> [V5]
  Demux/3 -> [V3]
  [P3c] -> Mux3/1
  Demux/1 -> [V1]
  Demux/2 -> [V2]
  [P1c] -> Mux1/1
  [P2c] -> Mux1/2
  Demux/6 -> [V6]
  [P6c] -> Mux5/2
  Demux/7 -> [V7]
  [P7c] -> Mux4/1
  Demux/8 -> [V8]
  [P8c] -> Mux4/2
  Demux/10 -> [V10]
  [P10c] -> Mux4/4
  Demux/12 -> [V12]
  [P12c] -> Sum6/2
  [Pe13] -> Sum7/1
  Demux/15 -> [V15]
  [P15c] -> Mux2/1
  Demux/16 -> [Vpa]
  Demux/17 -> [Vpv]
  [Ppac] -> Mux2/2
  [Ppvc] -> Mux2/3
  Demux/11 -> [uV11]

== system cv_model_50M/Design of Experiment/Switch Block ==
  In1 : Inport
  In2 : Inport  Port=2
  Null Signal : Constant  Value=0
  Switch : Switch  Criteria=u2 > Threshold  Threshold=0.5  SaturateOnIntegerOverflow=off  InputSameDT=off
  Switch Control : Constant
  Switch1 : Switch  Criteria=u2 > Threshold  Threshold=0.5  SaturateOnIntegerOverflow=off  InputSameDT=off
  Tilt Angle : Outport
  Speed : Outport  Port=2
  tag scope: Ctrl=global
  wires:
  Switch Control/1 -> [Ctrl], Switch1/2, Switch/2
  Null Signal/1 -> Switch1/1, Switch/3
  In1/1 -> Switch/1
  Switch/1 -> Tilt Angle/1
  Switch1/1 -> Speed/1
  In2/1 -> Switch1/3
